simulink model "Vergleich_linear_nichtlinear"  (R2021b)
settings: Solver=FixedStepAuto  StartTime=0.0  StopTime=25  FixedStep=1/1e4  RelTol=1e-3
undefined symbols (not defined in the file): A, B, C, C_buck, d, d_dyn, L_buck, S, T_c, x_Ruhe
settings Model: Creator=basti  LastModifiedBy=basti

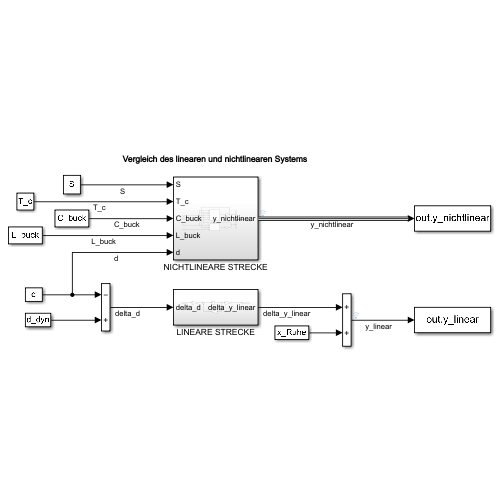
[thumbnail: Simulink's stored preview of the top-level diagram]
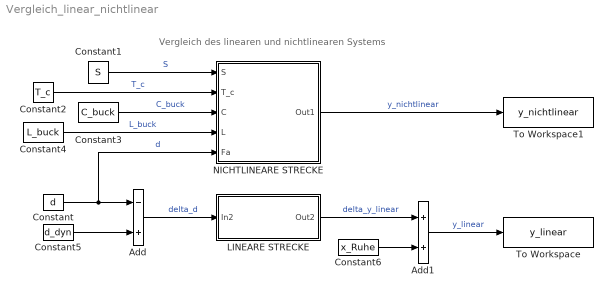
== system Vergleich_linear_nichtlinear ==
  note: Vergleich des linearen und nichtlinearen Systems
  Add : Sum  Inputs=-+
  Add1 : Sum
  Constant : Constant  Value=d
  Constant1 : Constant  Value=S
  Constant2 : Constant  Value=T_c
  Constant3 : Constant  Value=C_buck
  Constant4 : Constant  Value=L_buck
  Constant5 : Constant  Value=d_dyn
  Constant6 : Constant  Value=x_Ruhe
  LINEARE STRECKE : Subsystem
  NICHTLINEARE STRECKE : Subsystem
  To Workspace : ToWorkspace  VariableName=y_linear  SaveFormat=Timeseries  SampleTime=-1
  To Workspace1 : ToWorkspace  VariableName=y_nichtlinear  SaveFormat=Timeseries  SampleTime=-1
  wires:
  NICHTLINEARE STRECKE/1(Out1) -> To Workspace1/1  "y_nichtlinear"
  Constant1/1 -> NICHTLINEARE STRECKE/1(S)  "S"
  Constant2/1 -> NICHTLINEARE STRECKE/2(T_c)  "T_c"
  Constant4/1 -> NICHTLINEARE STRECKE/4(L)  "L_buck"
  Constant3/1 -> NICHTLINEARE STRECKE/3(C)  "C_buck"
  Constant/1 -> Add/1, NICHTLINEARE STRECKE/5(Fa)  "d"
  Constant5/1 -> Add/2
  Constant6/1 -> Add1/2
  Add1/1 -> To Workspace/1  "y_linear"
  LINEARE STRECKE/1(Out2) -> Add1/1  "delta_y_linear"
  Add/1 -> LINEARE STRECKE/1(In2)  "delta_d"

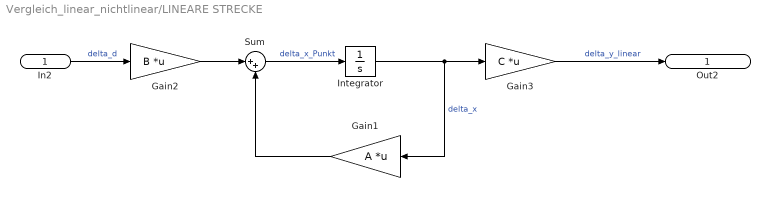
== system Vergleich_linear_nichtlinear/LINEARE STRECKE ==
  In2 : Inport
  Gain1 : Gain  Gain=A  Multiplication=Matrix(K*u) (u vector)
  Gain2 : Gain  Gain=B  Multiplication=Matrix(K*u) (u vector)
  Gain3 : Gain  Gain=C  Multiplication=Matrix(K*u) (u vector)
  Integrator : Integrator
  Sum : Sum  Inputs=|++
  Out2 : Outport
  wires:
  In2/1 -> Gain2/1  "delta_d"
  Gain2/1 -> Sum/1
  Gain1/1 -> Sum/2
  Sum/1 -> Integrator/1  "delta_x_Punkt"
  Integrator/1 -> Gain3/1, Gain1/1  "delta_x"
  Gain3/1 -> Out2/1  "delta_y_linear"

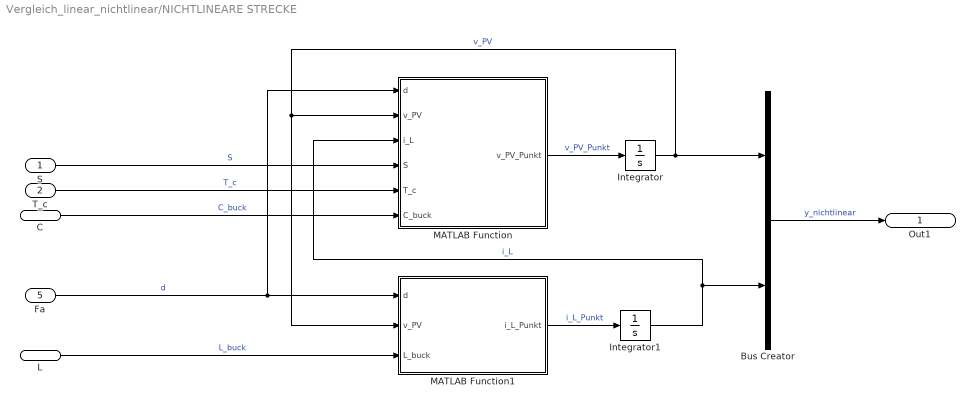
== system Vergleich_linear_nichtlinear/NICHTLINEARE STRECKE ==
  S : Inport
  T_c : Inport  Port=2
  C : Inport  Port=3
  L : Inport  Port=4
  Fa : Inport  Port=5
  Bus Creator : BusCreator  Inputs=2
  Integrator : Integrator
  Integrator1 : Integrator
  MATLAB Function : MATLAB Function  TreatAsAtomicUnit=on
  MATLAB Function1 : MATLAB Function  TreatAsAtomicUnit=on
  Out1 : Outport
  wires:
  MATLAB Function/1(v_PV_Punkt) -> Integrator/1  "v_PV_Punkt"
  MATLAB Function1/1(i_L_Punkt) -> Integrator1/1  "i_L_Punkt"
  Fa/1 -> MATLAB Function1/1(d), MATLAB Function/1(d)  "d"
  Bus Creator/1 -> Out1/1  "y_nichtlinear"
  Integrator1/1 -> MATLAB Function/3(i_L), Bus Creator/2  "i_L"
  Integrator/1 -> MATLAB Function/2(v_PV), MATLAB Function1/2(v_PV), Bus Creator/1  "v_PV"
  S/1 -> MATLAB Function/4(S)  "S"
  T_c/1 -> MATLAB Function/5(T_c)  "T_c"
  C/1 -> MATLAB Function/6(C_buck)  "C_buck"
  L/1 -> MATLAB Function1/3(L_buck)  "L_buck"

== matlab function Vergleich_linear_nichtlinear/NICHTLINEARE STRECKE/MATLAB Function1 ==
  data: d input; i_L_Punkt output; v_PV input; L_buck input
% EINGÄNGE
% d                 Duty Cycle
% v_PV              PV-Spannung
% L_buck            Induktivitätswert

% AUSGÄNGE
% i_L_Punkt        zeitliche Ableitung des Stroms i_L

function i_L_Punkt = fcn(d, v_PV, L_buck)
    % Konstanten
    c = Konstanten();

    % Berechnung
    i_L_Punkt = 1/L_buck * v_PV * d - 1/L_buck * c.v_DC;

== matlab function Vergleich_linear_nichtlinear/NICHTLINEARE STRECKE/MATLAB Function ==
  data: d input; v_PV_Punkt output; v_PV input; i_L input; S input; T_c input; C_buck input
% EINGÄNGE
% d                 Duty Cycle
% v_PV              PV-Spannung
% i_L               Strom i_L
% S                 Eingangsstrahlung
% T_c               Zellentemperatur
% C_buck            Kondensatorwert

% AUSGÄNGE
% v_PV_Punkt        zeitliche Ableitung der PV-Spannung

function v_PV_Punkt = fcn(d, v_PV, i_L, S, T_c, C_buck)
    % Konstanten
    c = Konstanten();

    % Berechnung
    v_oc = @(T_c) c.v_oc_STC * (1 + c.beta_T * (T_c - c.T_c_STC));                                      % für Modul
    i_ph = @(S, T_c) (S/c.S_STC) * c.i_ph_sc_STC * (1 + c.alpha_T * (T_c - c.T_c_STC));                 % für Modul
    i_s = @(S, T_c) (i_ph(S, T_c) - (v_oc(T_c)/c.R_h))/(exp(v_oc(T_c)/(c.A_n * c.v_T_STC)) - 1);        % für Modul
    i_d = @(x1, S, T_c) i_s(S, T_c) * (exp(x1/(c.N_s*c.v_T_STC * c.A_n)) - 1);                          % für Modul

    i_pv = @(x1, S, T_c) c.N_p * (i_ph(S, T_c) - i_d(x1, S, T_c) - x1/(c.N_s * c.R_h));

    v_PV_Punkt = 1/C_buck * i_pv(v_PV, S, T_c) - 1/C_buck * i_L * d;
